simulink model "TireModel"  (R2023b)
settings: Solver=VariableStepAuto  StartTime=0.0  StopTime=1  RelTol=1e-3
values from neighbouring files (symbols this model uses):
  c1 = 2/10    (= 0.2)    [TireModel_Parameters.m]
  c2 = 6628/1000    (= 6.628)    [TireModel_Parameters.m]
  c3 = 0    [TireModel_Parameters.m]
settings Model: Creator=BeanieBabyJ  LastModifiedBy=BeanieBabyJ

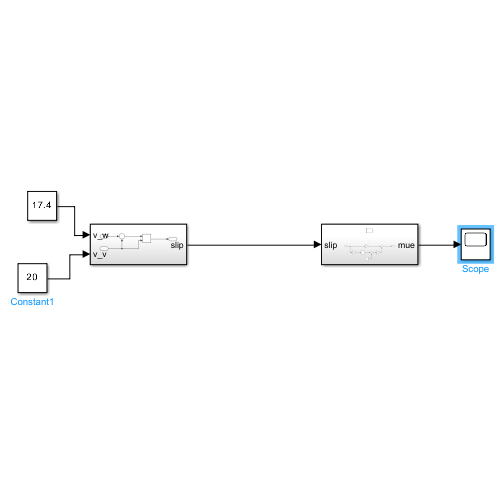
[thumbnail: Simulink's stored preview of the top-level diagram]
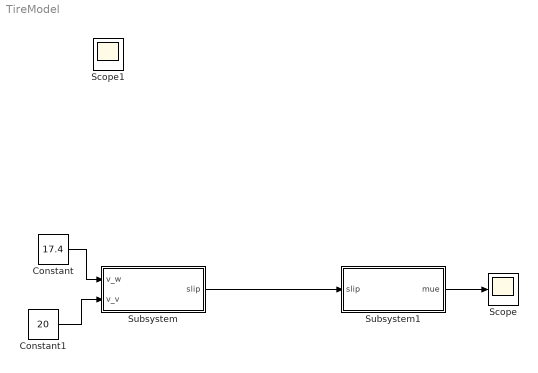
== system TireModel ==
  Constant : Constant  Value=17.4
  Constant1 : Constant  Value=20
  Scope : Scope
  Subsystem : Subsystem
  Subsystem1 : Subsystem
  Scope1 : Scope
  wires:
  Subsystem/1(slip) -> Subsystem1/1(slip)
  Subsystem1/1(mue) -> Scope/1
  Constant/1 -> Subsystem/1(v_w)
  Constant1/1 -> Subsystem/2(v_v)

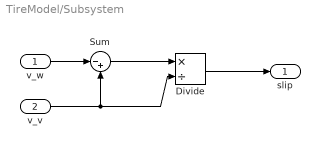
== system TireModel/Subsystem ==
  v_w : Inport
  v_v : Inport  Port=2
  Divide : Product  Inputs=*/
  Sum : Sum  Inputs=|-+
  slip : Outport
  wires:
  Sum/1 -> Divide/1
  v_v/1 -> Sum/2, Divide/2
  v_w/1 -> Sum/1
  Divide/1 -> slip/1

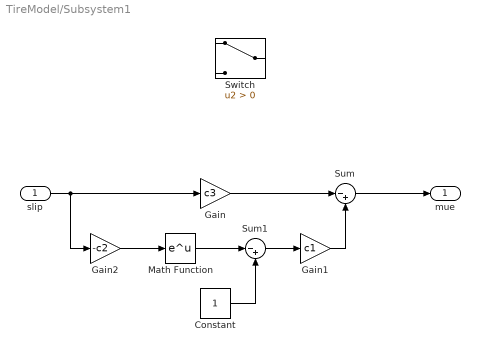
== system TireModel/Subsystem1 ==
  slip : Inport
  Constant : Constant
  Gain : Gain  Gain=c3
  Gain1 : Gain  Gain=c1
  Gain2 : Gain  Gain=-c2
  Math Function : Math
  Sum : Sum  Inputs=|-+
  Sum1 : Sum  Inputs=|-+
  Switch : Switch  Criteria=u2 > Threshold  SaturateOnIntegerOverflow=off  InputSameDT=off
  mue : Outport
  wires:
  Sum1/1 -> Gain1/1
  slip/1 -> Gain/1, Gain2/1
  Gain2/1 -> Math Function/1
  Math Function/1 -> Sum1/1
  Constant/1 -> Sum1/2
  Gain1/1 -> Sum/2
  Gain/1 -> Sum/1
  Sum/1 -> mue/1
